simulink model "Angle_FTVF_20a"  (R2021a)
settings: Solver=FixedStepAuto  StartTime=0.0  StopTime=10.0  RelTol=1e-3  EnableMultiTasking=on
libraries: arduinolib x6
settings Model: SILPILModeSetting=veronly  ExtModeTrigDuration=2  Creator=Siro  LastModifiedBy=david
settings OptimizationCC: EnhancedBackFolding=on  PassReuseOutputArgsAs=Individual arguments  ZeroExternalMemoryAtStartup=off  ZeroInternalMemoryAtStartup=off  MaxStackSize=64  OptimizeBlockOrder=speed  DifferentSizesBufferReuse=on  OptimizationCustomize=off  EfficientTunableParamExpr=on
settings DebuggingCC: ParameterTunabilityLossMsg=error
settings HardwareCC: ProdBitPerInt=16  ProdBitPerPointer=16  ProdBitPerSizeT=16  ProdBitPerPtrDiffT=16  ProdLargestAtomicFloat=None  ProdWordSize=8  ProdHWDeviceType=Atmel->AVR
settings SFSimCC: MATLABDynamicMemAlloc=off
settings RTWCC: SystemTargetFile=ert.tlc  HardwareBoard=Arduino Uno  TemplateMakefile=ert_default_tmf  Toolchain=Arduino AVR  BuildConfiguration=Faster Runs
settings CodeAppCC: ForceParamTrailComments=on  IgnoreCustomStorageClasses=off  OperatorAnnotations=on  SimulinkDataObjDesc=on  SFDataObjDesc=on  InsertBlockDesc=on
settings ERTTargetCC: SupportContinuousTime=on  SupportVariableSizeSignals=on  ExtModeStaticAllocSize=250

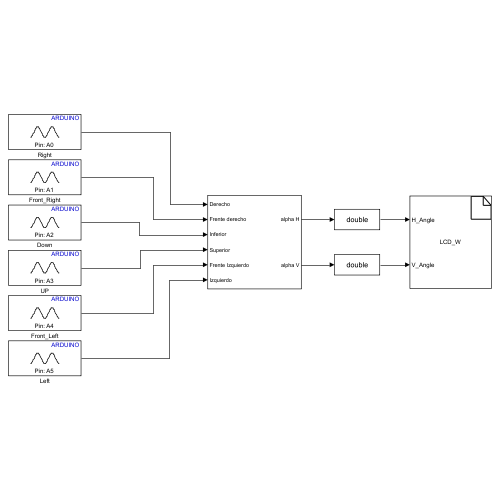
[thumbnail: Simulink's stored preview of the top-level diagram]
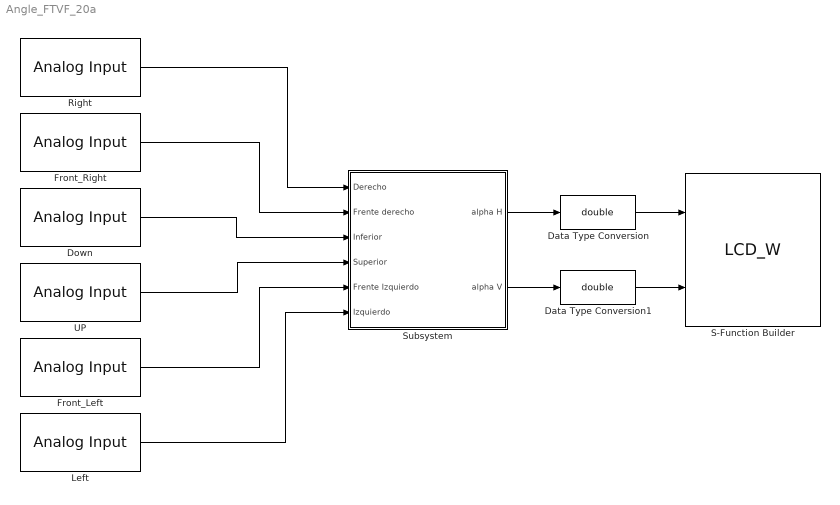
== system Angle_FTVF_20a ==
  Data Type Conversion : DataTypeConversion  OutDataTypeStr=double
  Data Type Conversion1 : DataTypeConversion  OutDataTypeStr=double
  Down : arduinolib/Analog Input  pinNumber=2  ReadResultsOnly=off  ConversionTriggerSource=Software  ExternalTriggerType=uint32( 0 )  OutputDataType=uint16  EnableConversionCompleteNotify=off  EnableOuputStatus=off  SampleTime=0.1  blockPlatform=arduino
  Front_Left : arduinolib/Analog Input  pinNumber=4  ReadResultsOnly=off  ConversionTriggerSource=Software  ExternalTriggerType=uint32( 0 )  OutputDataType=uint16  EnableConversionCompleteNotify=off  EnableOuputStatus=off  SampleTime=0.1  blockPlatform=arduino
  Front_Right : arduinolib/Analog Input  pinNumber=1  ReadResultsOnly=off  ConversionTriggerSource=Software  ExternalTriggerType=uint32( 0 )  OutputDataType=uint16  EnableConversionCompleteNotify=off  EnableOuputStatus=off  SampleTime=0.1  blockPlatform=arduino
  Left : arduinolib/Analog Input  pinNumber=5  ReadResultsOnly=off  ConversionTriggerSource=Software  ExternalTriggerType=uint32( 0 )  OutputDataType=uint16  EnableConversionCompleteNotify=off  EnableOuputStatus=off  SampleTime=0.1  blockPlatform=arduino
  Right : arduinolib/Analog Input  pinNumber=0  ReadResultsOnly=off  ConversionTriggerSource=Software  ExternalTriggerType=uint32( 0 )  OutputDataType=uint16  EnableConversionCompleteNotify=off  EnableOuputStatus=off  SampleTime=0.1  blockPlatform=arduino
  S-Function Builder : S-Function  FunctionName=LCD_W  SFunctionModules=LCD_W_wrapper  SFunctionDeploymentMode=off  EnableBusSupport=off  mask(S-Function Builder){}
      mask help: Simulink:masks:SFunctionBuilder_MD
      mask init:
      | val = [[.9  0.75 0.75 1 1 .9 .9 1]',[1 1 0.75 0.75 .9 .9 1 .9]'];try , sys = get_param(gcb,'SfunBuilderFcnName');if isempty(sys), sys = get_param(gcb,'FunctionName'); end,catch, sys = get_param(gcb,'FunctionName'); end
      settings: CopyFcn=set_param(gcbh,'LinkStatus','none')  OpenFcn=sfunctionwizard(gcbh)
      mask Display:
      | plot(val(:,1),val(:,2))
      | disp(sys)
      | port_label('input',1,'H_Angle')
      | port_label('input',2,'V_Angle')
  Subsystem : Subsystem
  UP : arduinolib/Analog Input  pinNumber=3  ReadResultsOnly=off  ConversionTriggerSource=Software  ExternalTriggerType=uint32( 0 )  OutputDataType=uint16  EnableConversionCompleteNotify=off  EnableOuputStatus=off  SampleTime=0.1  blockPlatform=arduino
  wires:
  Subsystem/2(alpha V) -> Data Type Conversion1/1
  Front_Right/1 -> Subsystem/2(Frente derecho)
  Down/1 -> Subsystem/3(Inferior)
  Front_Left/1 -> Subsystem/5(Frente Izquierdo)
  Subsystem/1(alpha H) -> Data Type Conversion/1
  Data Type Conversion/1 -> S-Function Builder/1
  UP/1 -> Subsystem/4(Superior)
  Left/1 -> Subsystem/6(Izquierdo)
  Right/1 -> Subsystem/1(Derecho)
  Data Type Conversion1/1 -> S-Function Builder/2

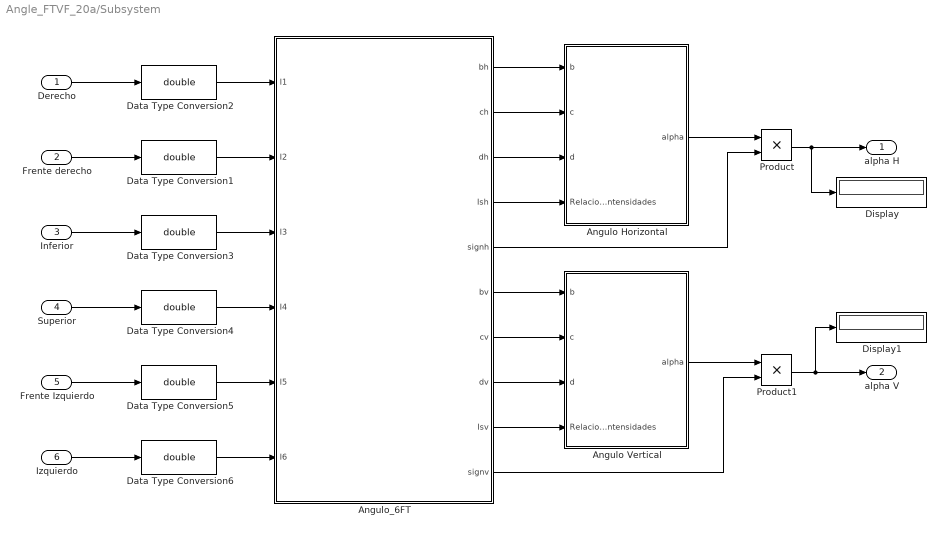
== system Angle_FTVF_20a/Subsystem ==
  Derecho : Inport
  Frente derecho : Inport  Port=2
  Inferior : Inport  Port=3
  Superior : Inport  Port=4
  Frente Izquierdo : Inport  Port=5
  Izquierdo : Inport  Port=6
  Angulo Horizontal : Subsystem
  Angulo Vertical : Subsystem
  Angulo_6FT : MATLAB Function  TreatAsAtomicUnit=on
  Data Type Conversion{1..6} (6 alike) : DataTypeConversion  OutDataTypeStr=double
  Display : Display
  Display1 : Display
  Product : Product
  Product1 : Product
  alpha H : Outport
  alpha V : Outport  Port=2
  wires:
  Data Type Conversion3/1 -> Angulo_6FT/3(I3)
  Angulo_6FT/8(dv) -> Angulo Vertical/3(d)
  Angulo_6FT/6(bv) -> Angulo Vertical/1(b)
  Product/1 -> alpha H/1, Display/1
  Angulo_6FT/7(cv) -> Angulo Vertical/2(c)
  Angulo Vertical/1(alpha) -> Product1/1
  Angulo_6FT/5(signh) -> Product/2
  Angulo_6FT/1(bh) -> Angulo Horizontal/1(b)
  Angulo_6FT/2(ch) -> Angulo Horizontal/2(c)
  Data Type Conversion5/1 -> Angulo_6FT/5(I5)
  Angulo_6FT/9(Isv) -> Angulo Vertical/4(Relacion de intensidades)
  Data Type Conversion2/1 -> Angulo_6FT/1(I1)
  Angulo_6FT/10(signv) -> Product1/2
  Data Type Conversion1/1 -> Angulo_6FT/2(I2)
  Data Type Conversion4/1 -> Angulo_6FT/4(I4)
  Data Type Conversion6/1 -> Angulo_6FT/6(I6)
  Angulo Horizontal/1(alpha) -> Product/1
  Product1/1 -> alpha V/1, Display1/1
  Angulo_6FT/3(dh) -> Angulo Horizontal/3(d)
  Angulo_6FT/4(Ish) -> Angulo Horizontal/4(Relacion de intensidades)
  Inferior/1 -> Data Type Conversion3/1
  Frente Izquierdo/1 -> Data Type Conversion5/1
  Izquierdo/1 -> Data Type Conversion6/1
  Derecho/1 -> Data Type Conversion2/1
  Frente derecho/1 -> Data Type Conversion1/1
  Superior/1 -> Data Type Conversion4/1

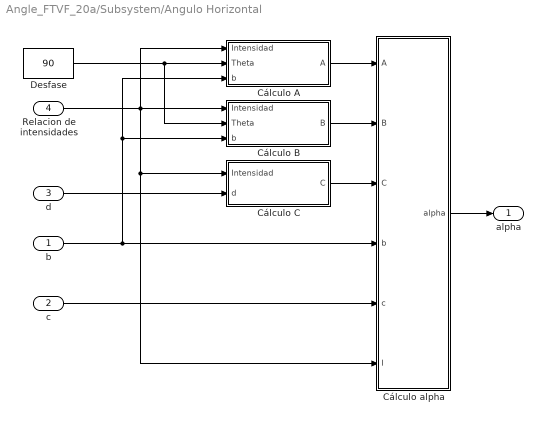
== system Angle_FTVF_20a/Subsystem/Angulo Horizontal ==
  b : Inport
  c : Inport  Port=2
  d : Inport  Port=3
  Relacion de intensidades : Inport  Port=4
  Cálculo A : Subsystem
  Cálculo B : Subsystem
  Cálculo C : Subsystem
  Cálculo alpha : MATLAB Function  TreatAsAtomicUnit=on
  Desfase : Constant  Value=90
  alpha : Outport
  wires:
  Cálculo alpha/1(alpha) -> alpha/1
  d/1 -> Cálculo C/2(d)
  Relacion de intensidades/1 -> Cálculo alpha/6(I), Cálculo C/1(Intensidad), Cálculo B/1(Intensidad), Cálculo A/1(Intensidad)
  b/1 -> Cálculo alpha/4(b), Cálculo B/3(b), Cálculo A/3(b)
  Cálculo C/1(C) -> Cálculo alpha/3(C)
  Cálculo B/1(B) -> Cálculo alpha/2(B)
  Cálculo A/1(A) -> Cálculo alpha/1(A)
  Desfase/1 -> Cálculo B/2(Theta), Cálculo A/2(Theta)
  c/1 -> Cálculo alpha/5(c)

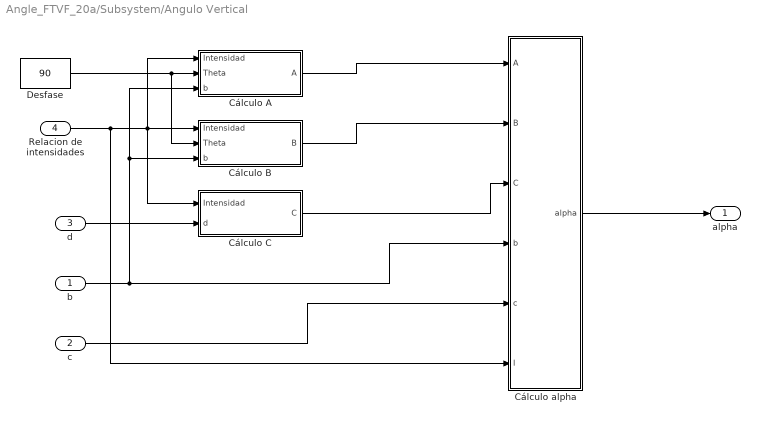
== system Angle_FTVF_20a/Subsystem/Angulo Vertical ==
  b : Inport
  c : Inport  Port=2
  d : Inport  Port=3
  Relacion de intensidades : Inport  Port=4
  Cálculo A : Subsystem
  Cálculo B : Subsystem
  Cálculo C : Subsystem
  Cálculo alpha : MATLAB Function  TreatAsAtomicUnit=on
  Desfase : Constant  Value=90
  alpha : Outport
  wires:
  Cálculo alpha/1(alpha) -> alpha/1
  d/1 -> Cálculo C/2(d)
  Relacion de intensidades/1 -> Cálculo alpha/6(I), Cálculo B/1(Intensidad), Cálculo A/1(Intensidad), Cálculo C/1(Intensidad)
  b/1 -> Cálculo alpha/4(b), Cálculo B/3(b), Cálculo A/3(b)
  Cálculo C/1(C) -> Cálculo alpha/3(C)
  Cálculo B/1(B) -> Cálculo alpha/2(B)
  Cálculo A/1(A) -> Cálculo alpha/1(A)
  Desfase/1 -> Cálculo B/2(Theta), Cálculo A/2(Theta)
  c/1 -> Cálculo alpha/5(c)

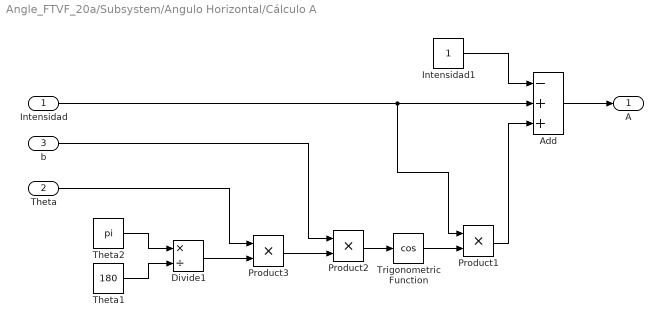
== system Angle_FTVF_20a/Subsystem/Angulo Horizontal/Cálculo A ==
  Intensidad : Inport
  Theta : Inport  Port=2
  b : Inport  Port=3
  Add : Sum  Inputs=-++
  Divide1 : Product  Inputs=*/
  Intensidad1 : Constant
  Product1 : Product
  Product2 : Product
  Product3 : Product
  Theta1 : Constant  Value=180
  Theta2 : Constant  Value=pi
  Trigonometric Function : Trigonometry  Operator=cos
  A : Outport
  wires:
  Divide1/1 -> Product3/2
  Product3/1 -> Product2/2
  Theta2/1 -> Divide1/1
  Intensidad1/1 -> Add/1
  Product1/1 -> Add/3
  Theta1/1 -> Divide1/2
  Trigonometric Function/1 -> Product1/2
  Product2/1 -> Trigonometric Function/1
  Intensidad/1 -> Product1/1, Add/2
  Theta/1 -> Product3/1
  Add/1 -> A/1
  b/1 -> Product2/1

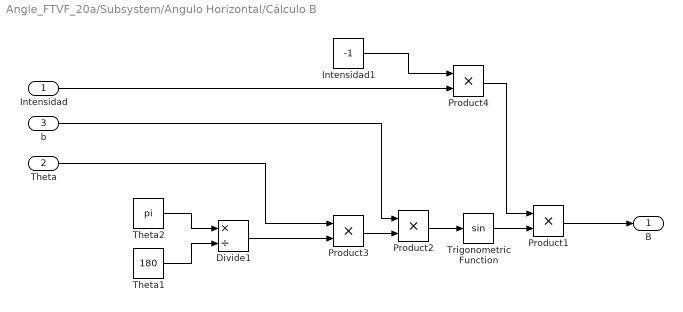
== system Angle_FTVF_20a/Subsystem/Angulo Horizontal/Cálculo B ==
  Intensidad : Inport
  Theta : Inport  Port=2
  b : Inport  Port=3
  Divide1 : Product  Inputs=*/
  Intensidad1 : Constant  Value=-1
  Product{1..4} (4 alike) : Product
  Theta1 : Constant  Value=180
  Theta2 : Constant  Value=pi
  Trigonometric Function : Trigonometry
  B : Outport
  wires:
  Divide1/1 -> Product3/2
  Product3/1 -> Product2/2
  Theta2/1 -> Divide1/1
  Product1/1 -> B/1
  Theta1/1 -> Divide1/2
  Trigonometric Function/1 -> Product1/2
  Product2/1 -> Trigonometric Function/1
  Intensidad/1 -> Product4/2
  Theta/1 -> Product3/1
  Intensidad1/1 -> Product4/1
  Product4/1 -> Product1/1
  b/1 -> Product2/1

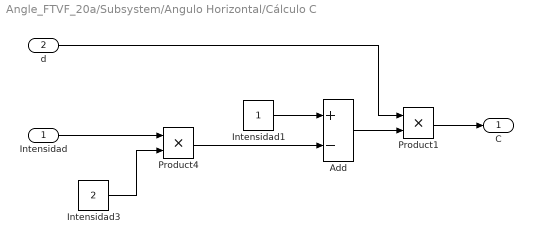
== system Angle_FTVF_20a/Subsystem/Angulo Horizontal/Cálculo C ==
  Intensidad : Inport
  d : Inport  Port=2
  Add : Sum  Inputs=+-
  Intensidad1 : Constant
  Intensidad3 : Constant  Value=2
  Product1 : Product
  Product4 : Product
  C : Outport
  wires:
  Intensidad1/1 -> Add/1
  Intensidad/1 -> Product4/1
  Intensidad3/1 -> Product4/2
  Product4/1 -> Add/2
  Add/1 -> Product1/2
  Product1/1 -> C/1
  d/1 -> Product1/1

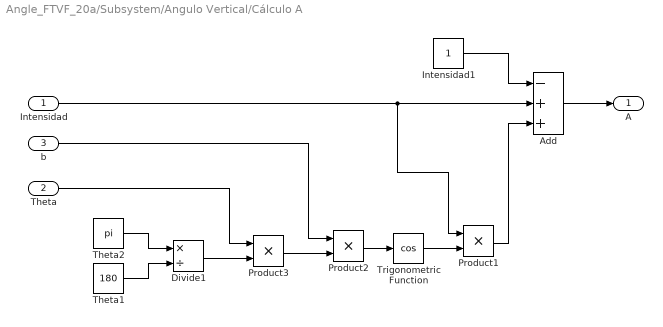
== system Angle_FTVF_20a/Subsystem/Angulo Vertical/Cálculo A ==
  Intensidad : Inport
  Theta : Inport  Port=2
  b : Inport  Port=3
  Add : Sum  Inputs=-++
  Divide1 : Product  Inputs=*/
  Intensidad1 : Constant
  Product1 : Product
  Product2 : Product
  Product3 : Product
  Theta1 : Constant  Value=180
  Theta2 : Constant  Value=pi
  Trigonometric Function : Trigonometry  Operator=cos
  A : Outport
  wires:
  Divide1/1 -> Product3/2
  Product3/1 -> Product2/2
  Theta2/1 -> Divide1/1
  Intensidad1/1 -> Add/1
  Product1/1 -> Add/3
  Theta1/1 -> Divide1/2
  Trigonometric Function/1 -> Product1/2
  Product2/1 -> Trigonometric Function/1
  Intensidad/1 -> Product1/1, Add/2
  Theta/1 -> Product3/1
  Add/1 -> A/1
  b/1 -> Product2/1

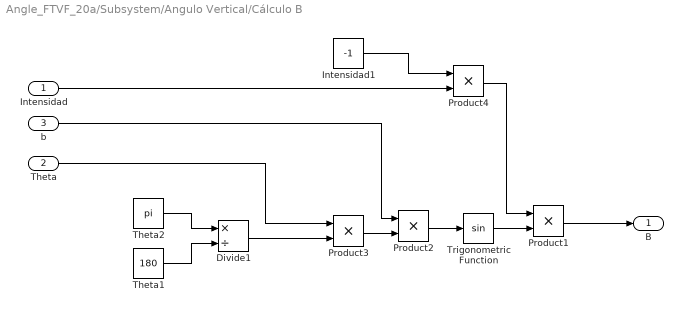
== system Angle_FTVF_20a/Subsystem/Angulo Vertical/Cálculo B ==
  Intensidad : Inport
  Theta : Inport  Port=2
  b : Inport  Port=3
  Divide1 : Product  Inputs=*/
  Intensidad1 : Constant  Value=-1
  Product{1..4} (4 alike) : Product
  Theta1 : Constant  Value=180
  Theta2 : Constant  Value=pi
  Trigonometric Function : Trigonometry
  B : Outport
  wires:
  Divide1/1 -> Product3/2
  Product3/1 -> Product2/2
  Theta2/1 -> Divide1/1
  Product1/1 -> B/1
  Theta1/1 -> Divide1/2
  Trigonometric Function/1 -> Product1/2
  Product2/1 -> Trigonometric Function/1
  Intensidad/1 -> Product4/2
  Theta/1 -> Product3/1
  Intensidad1/1 -> Product4/1
  Product4/1 -> Product1/1
  b/1 -> Product2/1

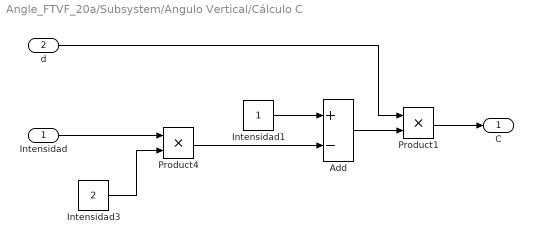
== system Angle_FTVF_20a/Subsystem/Angulo Vertical/Cálculo C ==
  Intensidad : Inport
  d : Inport  Port=2
  Add : Sum  Inputs=+-
  Intensidad1 : Constant
  Intensidad3 : Constant  Value=2
  Product1 : Product
  Product4 : Product
  C : Outport
  wires:
  Intensidad1/1 -> Add/1
  Intensidad/1 -> Product4/1
  Intensidad3/1 -> Product4/2
  Product4/1 -> Add/2
  Add/1 -> Product1/2
  Product1/1 -> C/1
  d/1 -> Product1/1

== matlab function Angle_FTVF_20a/Subsystem/Angulo Vertical/Cálculo alpha ==
  data: A input; alpha output; B input; C input; b input; c input; I input
function alpha = fcn(A, B, C, b, c,I)
    
    if ((I < 0.2) && (I > 0.8))
    alpha = 200;
    else
    if ((A+C ~= 0) && (-B*sqrt(A^2+B^2-C^2)+A^2+A*C+B^2 ~= 0))
        
        alpha = 2*atan((B-sqrt(A^2+B^2-C^2))/(A+C));

    elseif ((A+C ~= 0) && (B*sqrt(A^2+B^2-C^2)+A^2+A*C+B^2 ~= 0))

        alpha = 2*atan((B+sqrt(A^2+B^2-C^2))/(A+C));

    elseif ((B ~= 0) && (A^2+B^2~=0) && (C == -A))

        alpha = -2*atan(A/B);

    elseif (A == -C)

        alpha = pi;

    else

        alpha = 1000;

    end
    end
    alpha = (alpha -c*pi/180)/b;

    alpha = alpha*180/pi;

end

== matlab function Angle_FTVF_20a/Subsystem/Angulo_6FT ==
  data: I1 input; bh output; I2 input; I3 input; I4 input; I5 input; I6 input; ch output; dh output; Ish output; signh output; bv output; cv output; dv output; Isv output; signv output
function [bh,ch,dh,Ish,signh,bv,cv,dv,Isv,signv] = fcn(I1,I2,I3,I4,I5,I6)

%I1:Intensidad del FT derecho
%I2:Intensidad del FT frente/derecho
%I3:Intensidad del FT inferior
%I4:Intensidad del FT superior
%I5:Intensidad del FT frente/izquierdo
%I6:Intensidad del FT izquierdo

%bh: Coeficiente b para el ángulo horizontal
%ch: Coeficiente c para el ángulo horizontal
%dh: Coeficiente d para el ángulo horizontal
%ISH: Relación de intensidades para el ángulo horizontal
%signh: Signo del ángulo del plano horizontal

%bv: Coeficiente b para el ángulo vertical
%cv: Coeficiente c para el ángulo vertical
%dv: Coeficiente d para el ángulo vertical
%ISV: Relación de intensidades para el ángulo vertical
%signv: Signo del ángulo del plano vertical

%Plano Horizontal
if (((I1+1e-6)/(I6+1e-6) < 1.5) && ((I6+1e-6)/(I1+1e-6) < 1.5)) && ((I2>15)&&(I5>15)) % 0 
    bh = 1.7875;
    ch = 11.77375;
    dh = 1.57625;
    Ish = (cosd(11.77375 + 1.7875*0) + 1.57625)/(cosd(11.77375 + 1.7875*0) + 1.57625+cosd(11.77375 + 1.7875*90) + 1.57625);
    signh = 0; 
elseif I1 > I6 %0 - 90
    if (I1>I2)&&(((I6 > I2) && (I6 > I5)) || (((I2/(I5+1e-6) < 2.5) && (I5/(I2++1e-6) < 2.5)) && ((I2<10)||(I5<10)))) %90
        bh = 1;
        ch = 0;
        dh = 0;
        Ish = 0;
        signh = 1;
    else
        bh = 2.37125;
        ch = 2.827525;
        dh = 0.8898;
        Ish = I2/(I2+I1);
        signh = 1;
    end 
elseif I6 > I1 %0 - -90
    if (I6>I5)&&(((I1 > I2) && (I1 > I5)) || (((I2/(I5+1e-6) < 2.5)&&(I5/(I2+1e-6) < 2.5) )&& ((I2<15)||(I5<15)))) %-90
        bh = 1;
        ch = 0;
        dh = 0;
        Ish = 0;
        signh = -1;
    else
        bh = 2.316;
        ch = -21.4075;
        dh = 0.861975;
        Ish = I5/(I5+I6);
        signh = -1;  
    end
elseif (I1 <= 15)&&(I2 <= 5)&&(I5 <= 5)&&(I6 <= 15)%180
    bh = 1;
    ch = 0;
    dh = 0;
    Ish = 1;
    signh = 1;
else
    bh = 1;
    ch = 0;
    dh = 0;
    Ish = 1;
    signh = 0;    
end    
 
    
%Plano Vertical
if ((I3+1e-6)/(I4+1e-6) < 2) && ((I2+1e-6)/(I5+1e-6) < 2) % 0 
    bv = 1.7875;
    cv = 11.77375;
    dv = 1.57625;
    Isv = (cosd(11.77375 + 1.7875*0) + 1.57625)/(cosd(11.77375 + 1.7875*0) + 1.57625+cosd(11.77375 + 1.7875*90) + 1.57625);
    signv = 0;
elseif (I3 + 5 < I4)%0-90
    if ((I3 > I5)) || ((I5/I3 < 2.5) && (I3<10)) %90        
        bv = 1;
        cv = 0;
        dv = 0;
        Isv = 0;
        signv = 1;
    else
        bv = 1.7875;
        cv = 11.77375;
        dv = 1.57625;
        Isv = I5/(I4+I5);
        signv = 1;    
    end
elseif (I4 + 5< I3) %0- -90
    if ((I4 > I2)) || ((I2/I4 < 2.5) && (I4<10)) %-90        
        bv = 1;
        cv = 0;
        dv = 0;
        Isv = 0;
        signv = -1;
    else
        bv = 1.7875;
        cv = 11.77375;
        dv = 1.57625;
        Isv = I2/(I3+I2);
        signv = -1;    
    end
else
    bv = 1.7875;
    cv = 11.77375;
    dv = 1.57625;
    Isv = (cosd(11.77375 + 1.7875*0) + 1.57625)/(cosd(11.77375 + 1.7875*0) + 1.57625+cosd(11.77375 + 1.7875*90) + 1.57625);
    signv = 0;    
end

== matlab function Angle_FTVF_20a/Subsystem/Angulo Horizontal/Cálculo alpha ==
  data: A input; alpha output; B input; C input; b input; c input; I input
function alpha = fcn(A, B, C, b, c,I)
    
    if ((I < 0.2) && (I > 0.8))
    alpha = 200;
    else
    if ((A+C ~= 0) && (-B*sqrt(A^2+B^2-C^2)+A^2+A*C+B^2 ~= 0))
        
        alpha = 2*atan((B-sqrt(A^2+B^2-C^2))/(A+C));

    elseif ((A+C ~= 0) && (B*sqrt(A^2+B^2-C^2)+A^2+A*C+B^2 ~= 0))

        alpha = 2*atan((B+sqrt(A^2+B^2-C^2))/(A+C));

    elseif ((B ~= 0) && (A^2+B^2~=0) && (C == -A))

        alpha = -2*atan(A/B);

    elseif (A == -C)

        alpha = pi;

    else

        alpha = 1000;

    end
    end
    alpha = (alpha -c*pi/180)/b;

    alpha = alpha*180/pi;

end
